simulink model "simulink_example_v2017a"  (R2017a)
settings: Solver=VariableStepAuto  StartTime=0.0  StopTime=100  RelTol=1e-3
libraries: ProSivic_Sensors x4, simulink x1
settings Model: Creator=Markus Borg  LastModifiedBy=Markus Borg
settings DataIOCC: ReturnWorkspaceOutputs=on
settings SFSimCC: SimUseLocalCustomCode=on
settings RTWCC: RTWUseLocalCustomCode=on

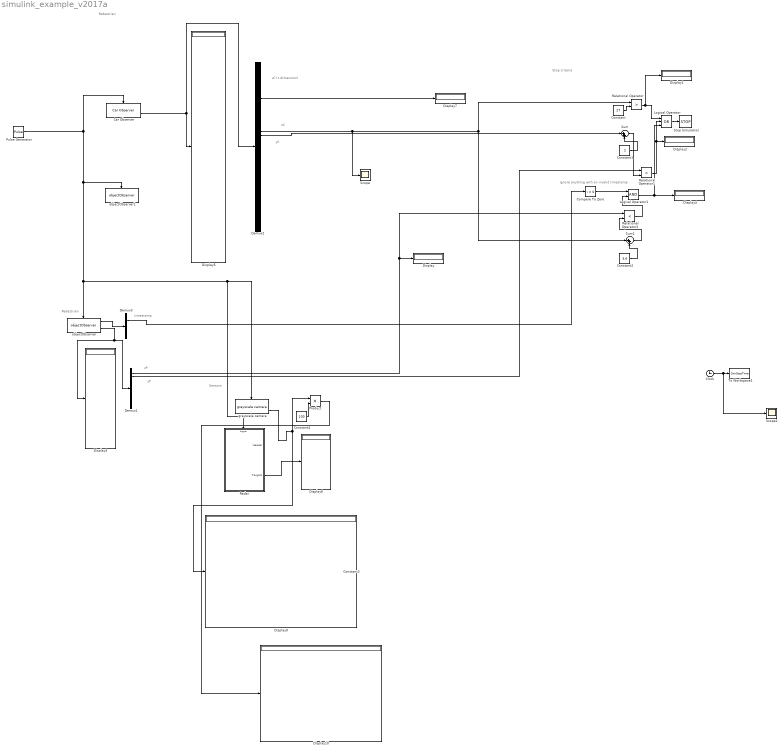
== system simulink_example_v2017a ==
  note: Stop criteria
  note: yP
  note: yC
  note: xP
  note: xC
  note: Pedestrian
  note: Sensors
  note: Pedestrian
  note: timestamp
  note: Ignore anything with an invalid timestamp
  note: vC (x dimension)
  " grayscale camera" : ProSivic_Sensors/ grayscale camera  topic=dashcam/cam  h=375  w=500  color=on
  Car Observer : ProSivic_Sensors/Car Observer  SystemSampleTime=-1
      link override S-Function: topic=egocar_obs/car_obs
  Clock : Clock
  Compare To Zero : simulink/Logic and Bit Operations/Compare To Zero  relop=~=  OutDataTypeStr=boolean
  Constant : Constant  Value=27
  Constant1 : Constant  Value=2
  Constant2 : Constant  Value=3.6
  Constant3 : Constant  Value=0
  Constant4 : Constant  Value=100
  Demux1 : Demux  Outputs=10
  Demux2 : Demux  Outputs=40
  Demux3 : Demux  Outputs=2
  Display{,1..7,9..10} (10 alike) : Display
  Logical Operator : Logic  Operator=OR  Inputs=3  AllPortsSameDT=off  OutDataTypeStr=boolean
  Logical Operator1 : Logic  AllPortsSameDT=off  OutDataTypeStr=boolean
  Product : Product  OutDataTypeStr=uint8
  Pulse Generator : DiscretePulseGenerator  PulseType=Time based  Period=0.005  PulseWidth=50
  Radar : Subsystem  Description=Radar block retreives the latest radar information from the ProSiVIC DDS store.  AncestorBlock=ProSivic_Sensors/Radar  TreatAsAtomicUnit=on
  Relational Operator : RelationalOperator  Operator=>  OutDataTypeStr=boolean  RndMeth=Simplest
  Relational Operator1 : RelationalOperator  Operator=>  OutDataTypeStr=boolean  RndMeth=Simplest
  Relational Operator2 : RelationalOperator  Operator=<  OutDataTypeStr=boolean  RndMeth=Simplest
  Scope : Scope
  Scope2 : Scope
  Stop Simulation : Stop
  Sum : Sum  Inputs=|++
  Sum1 : Sum  Inputs=|++
  To Workspace1 : ToWorkspace  VariableName=SimStopTime  SaveFormat=Structure With Time  SampleTime=-1
  objectObserver : ProSivic_Sensors/objectObserver  topic=ped_obs
  objectObserver1 : ProSivic_Sensors/objectObserver  topic=car_obj_obs
  wires:
  Pulse Generator/1 -> objectObserver/Trigger, " grayscale camera"/Trigger, Radar/Trigger, objectObserver1/Trigger, Car Observer/Trigger
  Relational Operator1/1 -> Display2/1, Logical Operator/2
  Demux1/1 -> Display/1, Relational Operator2/1
  Constant/1 -> Relational Operator/2
  objectObserver/2 -> Display3/1, Demux1/1
  Relational Operator/1 -> Display1/1, Logical Operator/1
  Constant1/1 -> Sum/2
  Demux1/2 -> Relational Operator1/1
  Constant2/1 -> Sum1/2
  Sum1/1 -> Relational Operator2/2
  Sum/1 -> Relational Operator1/2
  Logical Operator/1 -> Stop Simulation/1
  Car Observer/2 -> Demux2/1, Display5/1
  Demux2/16 -> Relational Operator/1, Sum1/1, Scope/1
  Demux2/17 -> Sum/1
  objectObserver/1 -> Demux3/1
  Demux3/1 -> Compare To Zero/1
  Compare To Zero/1 -> Logical Operator1/1
  Relational Operator2/1 -> Logical Operator1/2
  Logical Operator1/1 -> Logical Operator/3, Display4/1
  Clock/1 -> Scope2/1, To Workspace1/1
  Demux2/6 -> Display7/1
  Radar/2(Target1) -> Display6/1
  " grayscale camera"/2 -> Product/1, Display9/1
  Constant4/1 -> Product/2
  Product/1 -> Display10/1

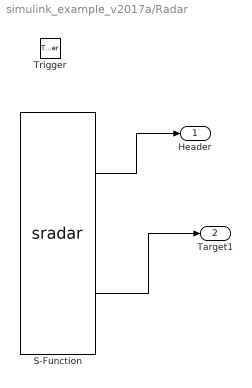
== system simulink_example_v2017a/Radar ==
  Trigger : TriggerPort  VariantControl=Variant
  S-Function : S-Function  FunctionName=sradar  Parameters=topic,nbmaxtarget  SFunctionDeploymentMode=off  EnableBusSupport=off  mask{topic=radar/radar, nbmaxtarget=1}
      mask prompts: topic "Radar Name"; nbmaxtarget "Number of targets"
  Header : Outport
  Target1 : Outport  Port=2
  wires:
  S-Function/2 -> Target1/1
  S-Function/1 -> Header/1
